simulink model "CalculatorUsingSubsystem"  (R2021a)
settings: Solver=FixedStepDiscrete  StartTime=0.0  StopTime=10.0  RelTol=1e-3
libraries: simulink x2
settings Model: Creator=OmarMedhat  LastModifiedBy=OmarMedhat
settings OptimizationCC: DefaultParameterBehavior=Inlined  EnhancedBackFolding=on  PassReuseOutputArgsAs=Individual arguments  ZeroExternalMemoryAtStartup=off  ZeroInternalMemoryAtStartup=off  OptimizeBlockOrder=speed  DifferentSizesBufferReuse=on  OptimizationCustomize=off  EfficientTunableParamExpr=on
settings DebuggingCC: ParameterTunabilityLossMsg=error
settings SFSimCC: MATLABDynamicMemAlloc=off
settings RTWCC: SystemTargetFile=ert.tlc  GenCodeOnly=on  TemplateMakefile=ert_default_tmf  GenerateReport=on  IncludeHyperlinkInReport=on  LaunchReport=on  GenerateTraceInfo=on
settings CodeAppCC: ForceParamTrailComments=on  IgnoreCustomStorageClasses=off  OperatorAnnotations=on  SimulinkDataObjDesc=on  SFDataObjDesc=on  InsertBlockDesc=on
settings ERTTargetCC: TargetLangStandard=C99 (ISO)  GenerateSampleERTMain=on  InlinedParameterPlacement=NonHierarchical  ERTCustomFileTemplate=example_file_process.tlc

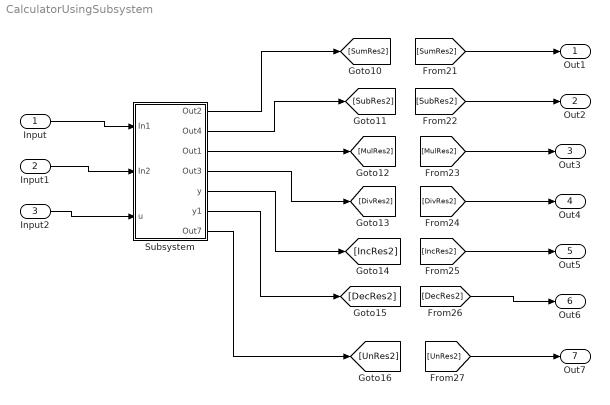
== system CalculatorUsingSubsystem ==
  Input : Inport
  Input1 : Inport  Port=2
  Input2 : Inport  Port=3
  Subsystem : Subsystem
  Out1 : Outport
  Out2 : Outport  Port=2
  Out3 : Outport  Port=3
  Out4 : Outport  Port=4
  Out5 : Outport  Port=5
  Out6 : Outport  Port=6
  Out7 : Outport  Port=7
  wires:
  [SubRes2] -> Out2/1
  Input1/1 -> Subsystem/2(In2)
  Input2/1 -> Subsystem/3(u)
  [DecRes2] -> Out6/1
  [SumRes2] -> Out1/1
  [UnRes2] -> Out7/1
  [MulRes2] -> Out3/1
  Input/1 -> Subsystem/1(In1)
  Subsystem/6(y1) -> [DecRes2]
  Subsystem/3(Out1) -> [MulRes2]
  Subsystem/2(Out4) -> [SubRes2]
  Subsystem/5(y) -> [IncRes2]
  Subsystem/4(Out3) -> [DivRes2]
  Subsystem/7(Out7) -> [UnRes2]
  [IncRes2] -> Out5/1
  Subsystem/1(Out2) -> [SumRes2]
  [DivRes2] -> Out4/1

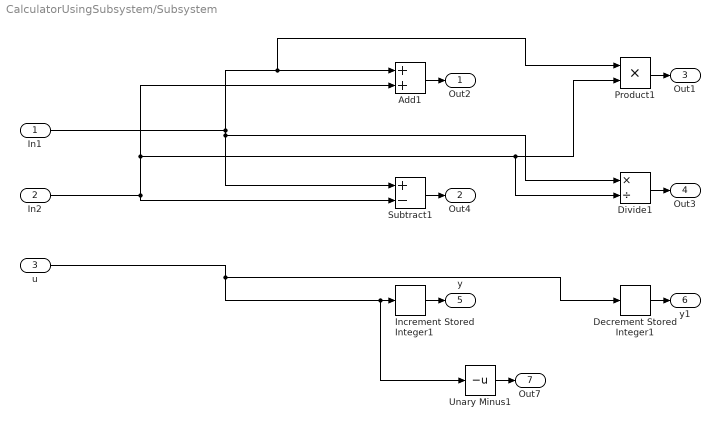
== system CalculatorUsingSubsystem/Subsystem ==
  In1 : Inport
  In2 : Inport  Port=2
  u : Inport  Port=3
  Add1 : Sum
  Decrement Stored Integer1 : simulink/Additional Math & Discrete/Additional Math: Increment - Decrement/Decrement Stored Integer
      settings: SourceProductBaseCode=SL
  Divide1 : Product  Inputs=*/
  Increment Stored Integer1 : simulink/Additional Math & Discrete/Additional Math: Increment - Decrement/Increment Stored Integer
  Product1 : Product
  Subtract1 : Sum  Inputs=+-
  Unary Minus1 : UnaryMinus
  Out2 : Outport
  Out4 : Outport  Port=2
  Out1 : Outport  Port=3
  Out3 : Outport  Port=4
  y : Outport  Port=5
  y1 : Outport  Port=6
  Out7 : Outport  Port=7
  wires:
  Increment Stored Integer1/1 -> y/1
  In2/1 -> Subtract1/2, Divide1/2, Product1/2, Add1/2
  In1/1 -> Product1/1, Add1/1, Subtract1/1, Divide1/1
  Divide1/1 -> Out3/1
  u/1 -> Decrement Stored Integer1/1, Unary Minus1/1, Increment Stored Integer1/1
  Subtract1/1 -> Out4/1
  Decrement Stored Integer1/1 -> y1/1
  Add1/1 -> Out2/1
  Unary Minus1/1 -> Out7/1
  Product1/1 -> Out1/1
